simulink model "SwcCELCmgr"  (R2017b)
settings: Solver=FixedStepDiscrete  StartTime=0.0  StopTime=50.0  RelTol=1e-3  EnableMultiTasking=on
libraries: simulink x1, CELCmgrLogicLib x1
settings Model: Creator=uidp6624  LastModifiedBy=Xiao Tao
settings DataIOCC: LimitDataPoints=on
settings OptimizationCC: DefaultParameterBehavior=Inlined  InlineInvariantSignals=on  BooleansAsBitfields=on  EnableMemcpy=off  StateBitsets=on  DataBitsets=on  ZeroExternalMemoryAtStartup=off  ZeroInternalMemoryAtStartup=off  NoFixptDivByZeroProtection=on  EfficientFloat2IntCast=on  LifeSpan=1
settings DebuggingCC: BusObjectLabelMismatch=error  SFUnexpectedBacktrackingDiag=warning  SFNoUnconditionalDefaultTransitionDiag=warning  SFExecutionAtInitializationDiag=none
settings HardwareCC: ProdBitPerPointer=32  ProdBitPerSizeT=32  ProdBitPerPtrDiffT=32  ProdLargestAtomicFloat=None  ProdWordSize=32  ProdHWDeviceType=Infineon->TriCore
settings ModelReferenceCC: PropagateSignalLabelsOutOfModel=off
settings SFSimCC: SimParseCustomCode=off  MATLABDynamicMemAlloc=off
settings RTWCC: SystemTargetFile=autosar.tlc  GenCodeOnly=on  TemplateMakefile=ert_default_tmf  Description=AUTOSAR  GenerateReport=on  BuildConfiguration=Faster Runs  IncludeHyperlinkInReport=on  LaunchReport=on  GenerateTraceInfo=on  GenerateTraceReport=on  GenerateTraceReportSl=on  GenerateTraceReportSf=on  GenerateTraceReportEml=on  GenerateCodeMetricsReport=on  GenerateCodeReplacementReport=on
settings CodeAppCC: ForceParamTrailComments=on  IgnoreCustomStorageClasses=off  OperatorAnnotations=on  SimulinkDataObjDesc=on  SFDataObjDesc=on  MATLABFcnDesc=on  InsertBlockDesc=on  StateflowObjectComments=on  MATLABSourceComments=on  ReqsInCode=on
settings STFCustomTargetCC: ParMdlRefBuildCompliant=on  CompOptLevelCompliant=on  IncludeMdlTerminateFcn=off  CombineOutputUpdateFcns=on  SuppressErrorStatus=on  ERTCustomFileBanners=on  SupportAbsoluteTime=off  SupportNonFinite=off  SupportComplex=off  PurelyIntegerCode=on  SupportContinuousTime=off  SupportNonInlinedSFcns=off  RemoveResetFunc=on  MATLABClassNameForMDSCustomization=Simulink.SoftwareTarget.ERTCustomization  AutosarCompliant=on  GRTInterface=off  UseToolchainInfoCompliant=on  LookupTableObjectStructAxisOrder=2,1,3,4,...  LUTObjectStructOrderEvenSpacing=Size,Table,Breakpoints  SystemTargetFile=autosar.tlc
settings ERTTargetCC: MultiwordLength=2048  ConcurrentExecutionCompliant=off  IncludeMdlTerminateFcn=off  SuppressErrorStatus=on  SupportAbsoluteTime=off  SupportNonFinite=off  SupportComplex=off  PurelyIntegerCode=on  ModelStepFunctionPrototypeControlCompliant=off  CPPClassGenCompliant=off  AutosarCompliant=on  LookupTableObjectStructAxisOrder=2,1,3,4,...  LUTObjectStructOrderEvenSpacing=Size,Table,Breakpoints  InlinedParameterPlacement=NonHierarchical  ERTCustomFileTemplate=example_file_process.tlc  GlobalDataReference=InSourceFile  ConvertIfToSwitch=off  SuppressUnreachableDefaultCases=off  EnableUserReplacementTypes=on  MemSecPackage=AUTOSAR  MemSecFuncInitTerm=SwAddrMethod  MemSecFuncExecute=SwAddrMethod  MemSecFuncSharedUtil=SwAddrMethod
settings ConfigComp: CovMetricSettings=dw  CovHtmlReporting=on  CovSaveCumulativeToWorkspaceVar=on  CovSaveSingleToWorkspaceVar=on  CovExternalEMLEnable=off

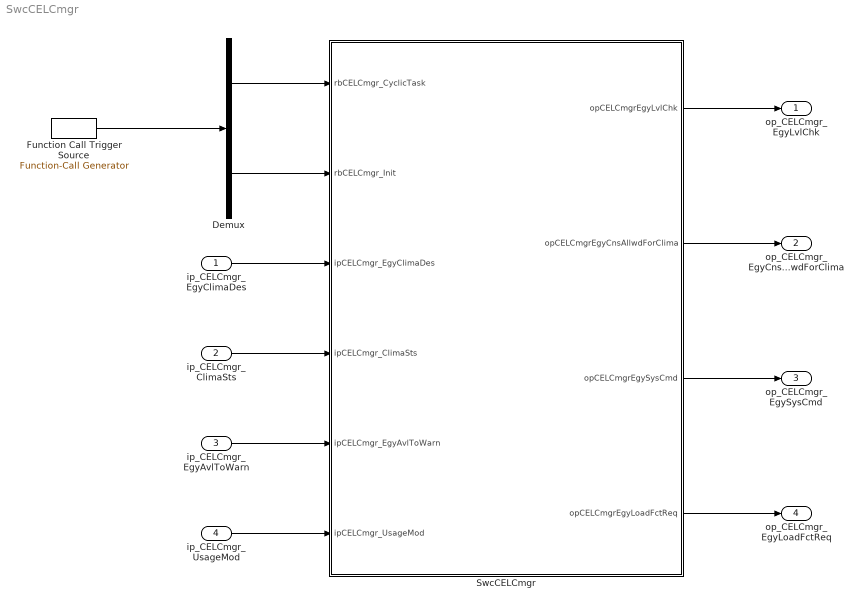
== system SwcCELCmgr ==
  ip_CELCmgr_EgyClimaDes : Inport  OutDataTypeStr=uint16  PortDimensions=1
  ip_CELCmgr_ClimaSts : Inport  Port=2  OutDataTypeStr=uint8  PortDimensions=1
  ip_CELCmgr_EgyAvlToWarn : Inport  Port=3  OutDataTypeStr=uint16  PortDimensions=1
  ip_CELCmgr_UsageMod : Inport  Port=4  OutDataTypeStr=uint8  PortDimensions=1
  Demux : Demux  Outputs=2
  Function Call Trigger Source : simulink/Ports & Subsystems/Function-Call Generator  sample_time=-1  numberOfIterations=1
  SwcCELCmgr : Subsystem
  op_CELCmgr_EgyLvlChk : Outport  OutDataTypeStr=uint8  PortDimensions=1
  op_CELCmgr_EgyCnsAllwdForClima : Outport  Port=2  OutDataTypeStr=uint16  PortDimensions=1
  op_CELCmgr_EgySysCmd : Outport  Port=3  OutDataTypeStr=uint8  PortDimensions=1
  op_CELCmgr_EgyLoadFctReq : Outport  Port=4  OutDataTypeStr=uint8  PortDimensions=1
  wires:
  Demux/2 -> SwcCELCmgr/2(rbCELCmgr_Init)
  Demux/1 -> SwcCELCmgr/1(rbCELCmgr_CyclicTask)
  Function Call Trigger Source/1 -> Demux/1
  ip_CELCmgr_EgyClimaDes/1 -> SwcCELCmgr/3(ipCELCmgr_EgyClimaDes)
  ip_CELCmgr_EgyAvlToWarn/1 -> SwcCELCmgr/5(ipCELCmgr_EgyAvlToWarn)
  ip_CELCmgr_ClimaSts/1 -> SwcCELCmgr/4(ipCELCmgr_ClimaSts)
  SwcCELCmgr/1(opCELCmgrEgyLvlChk) -> op_CELCmgr_EgyLvlChk/1
  SwcCELCmgr/2(opCELCmgrEgyCnsAllwdForClima) -> op_CELCmgr_EgyCnsAllwdForClima/1
  SwcCELCmgr/3(opCELCmgrEgySysCmd) -> op_CELCmgr_EgySysCmd/1
  ip_CELCmgr_UsageMod/1 -> SwcCELCmgr/6(ipCELCmgr_UsageMod)
  SwcCELCmgr/4(opCELCmgrEgyLoadFctReq) -> op_CELCmgr_EgyLoadFctReq/1

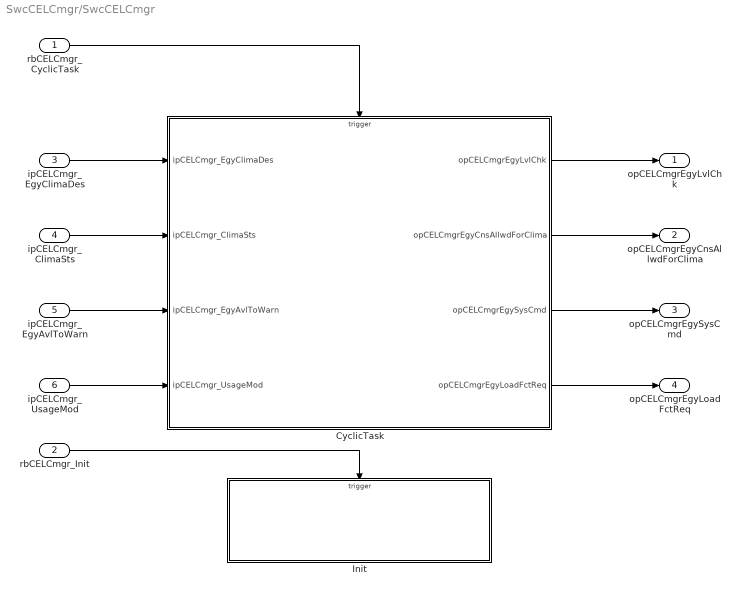
== system SwcCELCmgr/SwcCELCmgr ==
  rbCELCmgr_CyclicTask : Inport
  rbCELCmgr_Init : Inport  Port=2
  ipCELCmgr_EgyClimaDes : Inport  Port=3  OutDataTypeStr=uint16  PortDimensions=1
  ipCELCmgr_ClimaSts : Inport  Port=4  OutDataTypeStr=uint8  PortDimensions=1
  ipCELCmgr_EgyAvlToWarn : Inport  Port=5  OutDataTypeStr=uint16  PortDimensions=1
  ipCELCmgr_UsageMod : Inport  Port=6  OutDataTypeStr=uint8  PortDimensions=1
  CyclicTask : Subsystem  Description=Centralized energy load control function period task,T=10ms
  Init : Subsystem  Description=Centralized energy load control initialize function
  opCELCmgrEgyLvlChk : Outport  OutDataTypeStr=uint8  PortDimensions=1
  opCELCmgrEgyCnsAllwdForClima : Outport  Port=2  OutDataTypeStr=uint16  PortDimensions=1
  opCELCmgrEgySysCmd : Outport  Port=3  OutDataTypeStr=uint8  PortDimensions=1
  opCELCmgrEgyLoadFctReq : Outport  Port=4  OutDataTypeStr=uint8  PortDimensions=1
  wires:
  ipCELCmgr_EgyClimaDes/1 -> CyclicTask/1(ipCELCmgr_EgyClimaDes)
  rbCELCmgr_Init/1 -> Init/Trigger
  rbCELCmgr_CyclicTask/1 -> CyclicTask/Trigger
  ipCELCmgr_EgyAvlToWarn/1 -> CyclicTask/3(ipCELCmgr_EgyAvlToWarn)
  ipCELCmgr_UsageMod/1 -> CyclicTask/4(ipCELCmgr_UsageMod)
  CyclicTask/1(opCELCmgrEgyLvlChk) -> opCELCmgrEgyLvlChk/1
  CyclicTask/2(opCELCmgrEgyCnsAllwdForClima) -> opCELCmgrEgyCnsAllwdForClima/1
  CyclicTask/3(opCELCmgrEgySysCmd) -> opCELCmgrEgySysCmd/1
  CyclicTask/4(opCELCmgrEgyLoadFctReq) -> opCELCmgrEgyLoadFctReq/1
  ipCELCmgr_ClimaSts/1 -> CyclicTask/2(ipCELCmgr_ClimaSts)

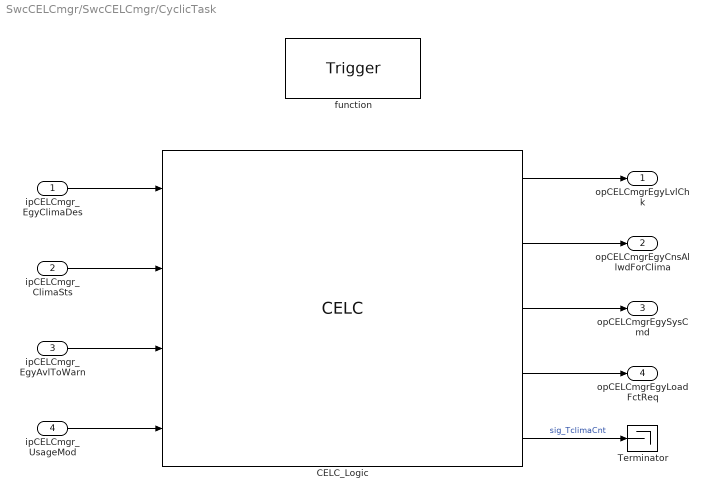
== system SwcCELCmgr/SwcCELCmgr/CyclicTask ==
  ipCELCmgr_EgyClimaDes : Inport  OutDataTypeStr=uint16  PortDimensions=1
  ipCELCmgr_ClimaSts : Inport  Port=2  OutDataTypeStr=uint8  PortDimensions=1
  ipCELCmgr_EgyAvlToWarn : Inport  Port=3  OutDataTypeStr=uint16  PortDimensions=1
  ipCELCmgr_UsageMod : Inport  Port=4  OutDataTypeStr=uint8  PortDimensions=1
  function : TriggerPort  TriggerType=function-call  VariantControl=Variant  PortDimensions=1
  CELC_Logic : CELCmgrLogicLib/CELC
  Terminator : Terminator
  opCELCmgrEgyLvlChk : Outport  OutDataTypeStr=uint8  PortDimensions=1
  opCELCmgrEgyCnsAllwdForClima : Outport  Port=2  OutDataTypeStr=uint16  PortDimensions=1
  opCELCmgrEgySysCmd : Outport  Port=3  OutDataTypeStr=uint8  PortDimensions=1
  opCELCmgrEgyLoadFctReq : Outport  Port=4  OutDataTypeStr=uint8  PortDimensions=1
  wires:
  ipCELCmgr_EgyAvlToWarn/1 -> CELC_Logic/3
  ipCELCmgr_EgyClimaDes/1 -> CELC_Logic/1
  ipCELCmgr_ClimaSts/1 -> CELC_Logic/2
  CELC_Logic/2 -> opCELCmgrEgyCnsAllwdForClima/1
  ipCELCmgr_UsageMod/1 -> CELC_Logic/4
  CELC_Logic/3 -> opCELCmgrEgySysCmd/1
  CELC_Logic/4 -> opCELCmgrEgyLoadFctReq/1
  CELC_Logic/5 -> Terminator/1  "sig_TclimaCnt"
  CELC_Logic/1 -> opCELCmgrEgyLvlChk/1

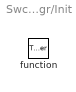
== system SwcCELCmgr/SwcCELCmgr/Init ==
  function : TriggerPort  TriggerType=function-call  VariantControl=Variant  PortDimensions=1
